simulink model "buck_boost_balance"  (R2024b)
settings: Solver=VariableStepAuto  StartTime=0.0  StopTime=2000  RelTol=1e-3
InitFcn:
  | M=0.1;
  | L=1;
  | T=1;
  | D=55;
undefined symbols (not defined in the file): Ion, Lithium
libraries: simulink x14, spsMosfetLib x14, spsBatteryLib x8, spsSeriesRLCBranchLib x7, spsControlledCurrentSourceLib x1, spsMultimeterLib x1, spspowerguiLib x1
settings Model: Creator=点墨  LastModifiedBy=32635
settings SolverCC: AlgebraicLoopSolver=TrustRegion
settings RTWCC: GPUComputeCapability=3.5

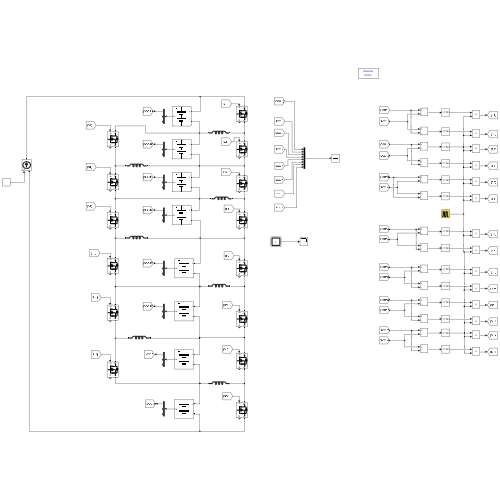
[thumbnail: Simulink's stored preview of the top-level diagram]
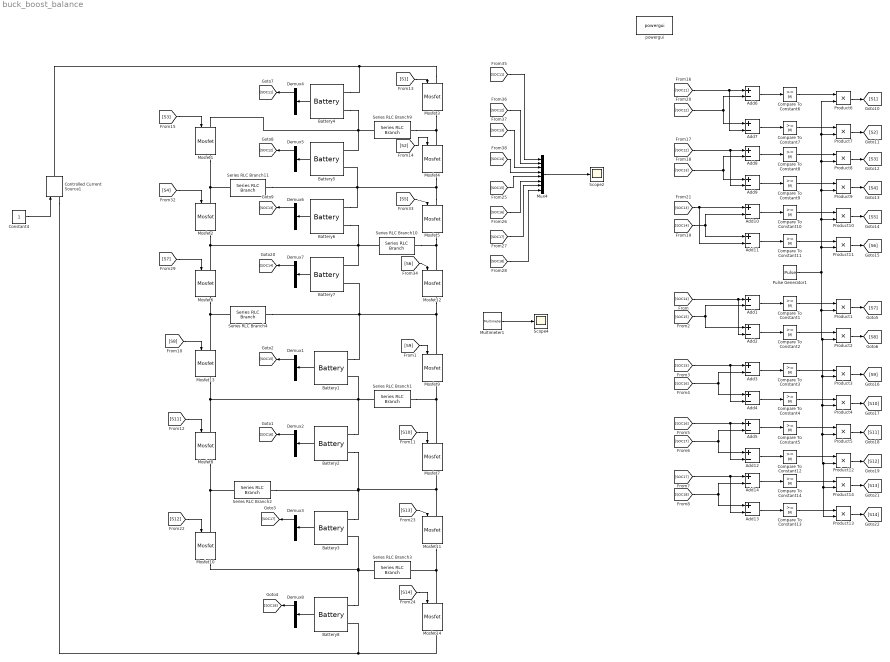
== system buck_boost_balance ==
  Add{1..14} (14 alike) : Sum  Inputs=+-
  Battery1 : spsBatteryLib/Battery  BatType=Lithium-Ion  NomV=3.2  NomQ=3.2  SOC=45  Batt_Tr=30  PresetModel=on  MaxQ=3.2  MinV=2.4  FullV=3.7248  Dis_rate=1.3913  R=0.01  Normal_OP=2.8939  expZone="[3.4572     0.15722]"
      settings: LibrarySourceBlock=electricdrivelib/Extra Sources/Battery
  Battery2 : spsBatteryLib/Battery  BatType=Lithium-Ion  NomV=3.2  NomQ=3.2  SOC=55  Batt_Tr=30  PresetModel=on  MaxQ=3.2  MinV=2.4  FullV=3.7248  Dis_rate=1.3913  R=0.01  Normal_OP=2.8939  expZone="[3.4572     0.15722]"
      settings: LibrarySourceBlock=electricdrivelib/Extra Sources/Battery
  Battery3 : spsBatteryLib/Battery  BatType=Lithium-Ion  NomV=3.2  NomQ=3.2  SOC=65  Batt_Tr=30  PresetModel=on  MaxQ=3.2  MinV=2.4  FullV=3.7248  Dis_rate=1.3913  R=0.01  Normal_OP=2.8939  expZone="[3.4572     0.15722]"
      settings: LibrarySourceBlock=electricdrivelib/Extra Sources/Battery
  Battery4 : spsBatteryLib/Battery  BatType=Lithium-Ion  NomV=3.2  NomQ=3.2  SOC=80  Batt_Tr=30  PresetModel=on  MaxQ=3.2  MinV=2.4  FullV=3.7248  Dis_rate=1.3913  R=0.01  Normal_OP=2.8939  expZone="[3.4572     0.15722]"
      settings: LibrarySourceBlock=electricdrivelib/Extra Sources/Battery
  Battery5 : spsBatteryLib/Battery  BatType=Lithium-Ion  NomV=3.2  NomQ=3.2  SOC=70  Batt_Tr=30  PresetModel=on  MaxQ=3.2  MinV=2.4  FullV=3.7248  Dis_rate=1.3913  R=0.01  Normal_OP=2.8939  expZone="[3.4572     0.15722]"
      settings: LibrarySourceBlock=electricdrivelib/Extra Sources/Battery
  Battery6 : spsBatteryLib/Battery  BatType=Lithium-Ion  NomV=3.2  NomQ=3.2  SOC=60  Batt_Tr=30  PresetModel=on  MaxQ=3.2  MinV=2.4  FullV=3.7248  Dis_rate=1.3913  R=0.01  Normal_OP=2.8939  expZone="[3.4572     0.15722]"
      settings: LibrarySourceBlock=electricdrivelib/Extra Sources/Battery
  Battery7 : spsBatteryLib/Battery  BatType=Lithium-Ion  NomV=3.2  NomQ=3.2  SOC=50  Batt_Tr=30  PresetModel=on  MaxQ=3.2  MinV=2.4  FullV=3.7248  Dis_rate=1.3913  R=0.01  Normal_OP=2.8939  expZone="[3.4572     0.15722]"
      settings: LibrarySourceBlock=electricdrivelib/Extra Sources/Battery
  Battery8 : spsBatteryLib/Battery  BatType=Lithium-Ion  NomV=3.2  NomQ=3.2  SOC=75  Batt_Tr=30  PresetModel=on  MaxQ=3.2  MinV=2.4  FullV=3.7248  Dis_rate=1.3913  R=0.01  Normal_OP=2.8939  expZone="[3.4572     0.15722]"
      settings: LibrarySourceBlock=electricdrivelib/Extra Sources/Battery
  Compare To Constant{1..14} (14 alike) : simulink/Logic and Bit Operations/Compare To Constant  relop=>=  const=M  OutDataTypeStr=boolean
  Constant4 : Constant
  Controlled Current Source1 : spsControlledCurrentSourceLib/Controlled Current Source  Initialize=on  Source_Type=DC  Amplitude=0  Phase=0  Frequency=0  Measurements=None
  Demux{1..8} (8 alike) : Demux  Outputs=3
  Mosfet{1..14} (14 alike) : spsMosfetLib/Mosfet  Ron=0.1  Lon=0  Rd=0.01  Vfd=0  IC=0  Rs=1e5  Cs=inf  Measurements=on
  Multimeter1 : spsMultimeterLib/Multimeter  L=3  sel=1  yselected={}  Gain=1  OutputType=Complex  PlotAtSimulationStop=off  PhasorSimulation=off
  Mux4 : Mux  Inputs=8
  Product{1..14} (14 alike) : Product
  Pulse Generator1 : DiscretePulseGenerator  PulseType=Time based  Period=T  PulseWidth=D
  Scope2 : Scope
  Scope4 : Scope
  Series RLC Branch1 : spsSeriesRLCBranchLib/Series RLC Branch  LConnTagsString=__new0  RConnTagsString=__new0  BranchType=L  Resistance=1  Inductance=L  SetiL0=off  InitialCurrent=0  Capacitance=1e-6  Setx0=off  InitialVoltage=0  Measurements=Branch current
  Series RLC Branch10 : spsSeriesRLCBranchLib/Series RLC Branch  LConnTagsString=__new0  RConnTagsString=__new0  BranchType=L  Resistance=1  Inductance=L  SetiL0=off  InitialCurrent=0  Capacitance=1e-6  Setx0=off  InitialVoltage=0  Measurements=Branch current
  Series RLC Branch{2,4,9,11} (4 alike) : spsSeriesRLCBranchLib/Series RLC Branch  LConnTagsString=__new0  RConnTagsString=__new0  BranchType=L  Resistance=1  Inductance=L  SetiL0=off  InitialCurrent=0  Capacitance=1e-6  Setx0=off  InitialVoltage=0  Measurements=None
  Series RLC Branch3 : spsSeriesRLCBranchLib/Series RLC Branch  LConnTagsString=__new0  RConnTagsString=__new0  BranchType=L  Resistance=1  Inductance=L  SetiL0=off  InitialCurrent=0  Capacitance=1e-6  Setx0=off  InitialVoltage=0  Measurements=Branch current
  powergui : spspowerguiLib/powergui  Priority=1  SimulationMode=Discrete  SampleTime=5e-2  frequency=60  Iterations=50  frequencyindice=0  Pbase=100e6  ErrMax=1e-4  UnitsV=kV  UnitsW=MW  buscounter=0  FunctionMessages=off  echomessages=off  EnableUseOfTLC=off  CurrentSourceSwitches=off  DisableSnubberDevices=off  DisableRonSwitches=off  DisableVfSwitches=off  DisplayEquations=off  AutomaticDiscreteSolvers=off  SolverType=Tustin/Backward Euler (TBE)  Interpol=off  ExternalGateDelay=off  methode=off  Ts=100  x0status=blocks  SPID=on  SwTol=0  HookPort=off  NonlinearTolerance=1e-4  nMaxIteration=100  ContinueOnMaxIteration=off  RestoreLinks=warning  ResistiveCurrentMeasurement=off  Frange=[0:2:500]  Ylog=off  Xlog=on  ShowGrid=off  save=off  variable=ZData  structure=0  ZoomFFT=off  StartTime=0.0  cycles=1  DisplayStyle=1  fundamental=60  FreqAxis=off  MaxFrequency=1000  frequencyindicesteady=1  RmsSteady=1  display=off
  wires:
  Compare To Constant11/1 -> Product11/1
  Add9/1 -> Compare To Constant9/1
  [SOC13] -> Add9/1, Add8/2
  Pulse Generator1/1 -> Product14/2, Product13/2, Product12/2, Product5/2, Product4/2, Product3/2, Product2/2, Product1/2, Product11/2, Product10/2, Product9/2, Product8/2, Product7/2, Product6/2
  [SOC13] -> Add11/2, Add10/1
  Add7/1 -> Compare To Constant7/1
  [SOC11] -> Add7/2, Add6/1
  Product6/1 -> [S1]
  Add6/1 -> Compare To Constant6/1
  Compare To Constant6/1 -> Product6/1
  Product10/1 -> [S5]
  Product8/1 -> [S3]
  Product11/1 -> [S6]
  Add10/1 -> Compare To Constant10/1
  Product9/1 -> [S4]
  [SOC12] -> Add7/1, Add6/2
  Constant4/1 -> Controlled Current Source1/1
  Add11/1 -> Compare To Constant11/1
  [S4] -> Mosfet2/1
  Multimeter1/1 -> Scope4/1
  Product7/1 -> [S2]
  Battery6/1 -> Demux6/1
  [S3] -> Mosfet1/1
  Battery5/1 -> Demux5/1
  [S2] -> Mosfet4/1
  [S5] -> Mosfet5/1
  [SOC11] -> Mux4/1
  Battery7/1 -> Demux7/1
  Demux5/1 -> [SOC12]
  Demux6/1 -> [SOC13]
  [SOC12] -> Add9/2, Add8/1
  Compare To Constant8/1 -> Product8/1
  [S6] -> Mosfet12/1
  Add8/1 -> Compare To Constant8/1
  Battery4/1 -> Demux4/1
  Compare To Constant9/1 -> Product9/1
  Demux7/1 -> [SOC14]
  [SOC12] -> Mux4/2
  [SOC13] -> Mux4/3
  Mux4/1 -> Scope2/1
  [S1] -> Mosfet3/1
  Compare To Constant7/1 -> Product7/1
  [SOC14] -> Mux4/4
  Compare To Constant10/1 -> Product10/1
  [SOC14] -> Add10/2, Add11/1
  Demux4/1 -> [SOC11]
  [S9] -> Mosfet9/1
  Demux1/1 -> [SOC15]
  Battery1/1 -> Demux1/1
  Battery2/1 -> Demux2/1
  Demux2/1 -> [SOC16]
  Battery3/1 -> Demux3/1
  Demux3/1 -> [SOC17]
  Battery8/1 -> Demux8/1
  Demux8/1 -> [SOC18]
  Add1/1 -> Compare To Constant1/1
  Add2/1 -> Compare To Constant2/1
  [SOC15] -> Add1/2, Add2/1
  [SOC14] -> Add2/2, Add1/1
  Compare To Constant1/1 -> Product1/1
  Compare To Constant2/1 -> Product2/1
  [SOC15] -> Add4/2, Add3/1
  Compare To Constant3/1 -> Product3/1
  Add3/1 -> Compare To Constant3/1
  [SOC16] -> Add3/2, Add4/1
  Compare To Constant4/1 -> Product4/1
  Add4/1 -> Compare To Constant4/1
  [SOC16] -> Add12/2, Add5/1
  Compare To Constant5/1 -> Product5/1
  Add5/1 -> Compare To Constant5/1
  [SOC17] -> Add5/2, Add12/1
  Compare To Constant12/1 -> Product12/1
  Add12/1 -> Compare To Constant12/1
  Compare To Constant13/1 -> Product13/1
  Compare To Constant14/1 -> Product14/1
  [SOC17] -> Add13/2, Add14/1
  [SOC18] -> Add14/2, Add13/1
  Add14/1 -> Compare To Constant14/1
  Add13/1 -> Compare To Constant13/1
  Product1/1 -> [S7]
  Product2/1 -> [S8]
  Product3/1 -> [S9]
  Product4/1 -> [S10]
  Product5/1 -> [S11]
  Product12/1 -> [S12]
  Product14/1 -> [S13]
  Product13/1 -> [S14]
  [S8] -> Mosfet13/1
  [S10] -> Mosfet7/1
  [S13] -> Mosfet11/1
  [S14] -> Mosfet14/1
  [SOC15] -> Mux4/5
  [SOC16] -> Mux4/6
  [SOC18] -> Mux4/8
  [SOC17] -> Mux4/7
  [S7] -> Mosfet6/1
  [S11] -> Mosfet8/1
  [S12] -> Mosfet10/1
  connections:
  Mosfet3/LConn1 -- Battery4/LConn1 -- Controlled Current Source1/RConn1
  Mosfet5/RConn1 -- Series RLC Branch10/LConn1 -- Mosfet12/LConn1
  Mosfet3/RConn1 -- Series RLC Branch9/LConn1 -- Mosfet4/LConn1
  Series RLC Branch9/RConn1 -- Battery5/LConn1 -- Battery4/LConn2 -- Mosfet1/LConn1
  Mosfet1/RConn1 -- Series RLC Branch11/LConn1 -- Mosfet2/LConn1
  Mosfet5/LConn1 -- Series RLC Branch11/RConn1 -- Battery5/LConn2 -- Battery6/LConn1 -- Mosfet4/RConn1
  Mosfet2/RConn1 -- Mosfet6/LConn1 -- Series RLC Branch10/RConn1 -- Battery7/LConn1 -- Battery6/LConn2
  Battery7/LConn2 -- Series RLC Branch4/RConn1 -- Mosfet9/LConn1 -- Mosfet12/RConn1 -- Battery1/LConn1
  Mosfet13/RConn1 -- Mosfet8/LConn1 -- Battery2/LConn1 -- Series RLC Branch1/RConn1 -- Battery1/LConn2
  Series RLC Branch4/LConn1 -- Mosfet6/RConn1 -- Mosfet13/LConn1
  Series RLC Branch1/LConn1 -- Mosfet7/LConn1 -- Mosfet9/RConn1
  Battery2/LConn2 -- Series RLC Branch2/RConn1 -- Battery3/LConn1 -- Mosfet11/LConn1 -- Mosfet7/RConn1
  Mosfet8/RConn1 -- Mosfet10/LConn1 -- Series RLC Branch2/LConn1
  Mosfet10/RConn1 -- Battery8/LConn1 -- Series RLC Branch3/RConn1 -- Battery3/LConn2
  Mosfet11/RConn1 -- Mosfet14/LConn1 -- Series RLC Branch3/LConn1
  Mosfet14/RConn1 -- Battery8/LConn2 -- Controlled Current Source1/LConn1
